simulink library "Lib_Piccolo"  (R2018b)
settings: Solver=VariableStepAuto  StartTime=0.0  StopTime=10.0  RelTol=1e-3
values from neighbouring files (symbols this model uses):
  AccelErrInt2Brakes = 0.15    [SimulationControlConfig16P.m]    (also in SimulationControlConfig16P_F0.m; SimulationControlConfig16P_F2.m; SimulationControlConfig16P_LEGACY.m; SimulationControlConfigTAILLESS.m = 0.2)
  AileronMax = 25    [SimulationControlConfig16P.m]    (also in SimulationControlConfig16P_F0.m; SimulationControlConfig16P_F2.m; SimulationControlConfig16P_LEGACY.m; SimulationControlConfigTAILLESS.m)
  AileronPower = 0.00268    [SimulationControlConfig16P.m]    (also in SimulationControlConfig16P_F0.m; SimulationControlConfig16P_F2.m; SimulationControlConfig16P_LEGACY.m; SimulationControlConfigTAILLESS.m = 0.002266)
  AileronSurfaceMax = 45    [SimulationControlConfig16P.m]    (also in SimulationControlConfig16P_F0.m; SimulationControlConfig16P_F2.m; SimulationControlConfig16P_LEGACY.m; SimulationControlConfigTAILLESS_CGAFT_F0.m = 25)
  AileronTrim = 0    [SimulationControlConfig16P.m]    (also in SimulationControlConfig16P_F0.m; SimulationControlConfig16P_F2.m; SimulationControlConfig16P_LEGACY.m; SimulationControlConfigTAILLESS.m)
  Alt = 1000 + TerrainHeight    [SimulationStateConfig.m]
  AltCruise_m = Alt * 0.3048    [SimulationControlConfig16P.m]    (also in SimulationControlConfig16P_F2.m; SimulationControlConfigTAILLESS.m = Alt/3.28084; SimulationControlConfigTAILLESS_CGAFT_F0.m = 640; SimulationControlConfigTAILLESS_CGFWD_F0.m = 640)
  AltitudeRate2PitchCmdIntegratorInit = 0.1    [SimulationControlPre.m]
  AltMax = 10000    [SimulationControlConfig16P.m]    (also in SimulationControlConfig16P_F0.m; SimulationControlConfig16P_F2.m; SimulationControlConfig16P_LEGACY.m; SimulationControlConfigTAILLESS.m)
  AltMaxAccel = 2.5    [SimulationControlConfig16P.m]    (also in SimulationControlConfig16P_F0.m = 2; SimulationControlConfig16P_F2.m = 2; SimulationControlConfig16P_LEGACY.m = 0.9; SimulationControlConfigTAILLESS.m = 2)
  AltMin = 0    [SimulationControlConfig16P.m]    (also in SimulationControlConfig16P_F0.m; SimulationControlConfig16P_F2.m; SimulationControlConfig16P_LEGACY.m; SimulationControlConfigTAILLESS.m)
  AltRateCmd2Pitch = 0.26    [SimulationControlConfig16P.m]    (also in SimulationControlConfig16P_F0.m = 0.35; SimulationControlConfig16P_F2.m = 0.35; SimulationControlConfig16P_LEGACY.m = 0.6; SimulationControlConfigTAILLESS.m = 0.9)
  AltRateError2Pitch = 0.34    [SimulationControlConfig16P.m]    (also in SimulationControlConfig16P_F0.m = 0.61; SimulationControlConfig16P_F2.m = 0.61; SimulationControlConfig16P_LEGACY.m = 0.4; SimulationControlConfigTAILLESS.m = 0.3)
  AltRateErrorInt2Pitch = 0.61    [SimulationControlConfig16P.m]    (also in SimulationControlConfig16P_F0.m = 0.28; SimulationControlConfig16P_F2.m = 0.28; SimulationControlConfig16P_LEGACY.m = 0.45; SimulationControlConfigTAILLESS.m = 0.15)
  AltRateLpfCutOff = 3    [SimulationControlConfig16P.m]    (also in SimulationControlConfig16P_F0.m; SimulationControlConfig16P_F2.m; SimulationControlConfig16P_LEGACY.m; SimulationControlConfigTAILLESS.m = 5)
  AutoNosegear2Rudder = 26    [SimulationControlConfig16P.m]    (also in SimulationControlConfig16P_F0.m; SimulationControlConfig16P_F2.m; SimulationControlConfig16P_LEGACY.m; SimulationControlConfigTAILLESS.m = 25.2)
  b = 5.54    [SimulationControlConfig16P.m]    (also in SimulationControlConfig16P_F0.m; SimulationControlConfig16P_F2.m; SimulationControlConfig16P_LEGACY.m; SimulationControlConfigTAILLESS.m = 2.37)
  Bank2AileronIntegratorInit = 0    [SimulationControlPre.m]
  BankMax_User = BankMax_User/180*pi    (= 0.610865238198)    [SimulationControlConfig16P.m]    (also in SimulationControlConfig16P_F0.m = 0.523598775598; SimulationControlConfig16P_F2.m = 0.523598775598; SimulationControlConfig16P_LEGACY.m = 0.523598775598; SimulationControlConfigTAILLESS.m = 0.558505360638)
  baseLegFlaps = 20    [SimulationControlConfig16P.m]    (also in SimulationControlConfig16P_F0.m; SimulationControlConfig16P_F2.m = 15; SimulationControlConfig16P_LEGACY.m = 0; SimulationControlConfigTAILLESS.m = 0)
  C = GeneticOpt.C    [SimulationCostFunction.m]
  c = Sw/b    (= 0.841696750903)    [SimulationControlConfig16P.m]    (also in SimulationControlConfig16P_F0.m; SimulationControlConfig16P_F2.m; SimulationControlConfig16P_LEGACY.m; SimulationControlConfigTAILLESS.m = 0.354008438819)
  cell2WheelFactorMG = 5.98    [SimulationSensorConfig16P_LEGACY.m]
  cell2WheelFactorNG = 1    [SimulationSensorConfig16P_LEGACY.m]
  cellSatMaxMG = 15000    [SimulationSensorConfig16P.m]    (also in SimulationSensorConfig16P_LEGACY.m; SimulationSensorConfigTAILLESS7P.m; SimulationSensorConfigUTAIL7P.m)
  cellSatMaxNG = 1000    [SimulationSensorConfig16P.m]    (also in SimulationSensorConfig16P_LEGACY.m; SimulationSensorConfigTAILLESS7P.m; SimulationSensorConfigUTAIL7P.m)
  cellSatMinMG = -15000    [SimulationSensorConfig16P.m]    (also in SimulationSensorConfig16P_LEGACY.m; SimulationSensorConfigTAILLESS7P.m; SimulationSensorConfigUTAIL7P.m)
  cellSatMinNG = -1000    [SimulationSensorConfig16P.m]    (also in SimulationSensorConfig16P_LEGACY.m; SimulationSensorConfigTAILLESS7P.m; SimulationSensorConfigUTAIL7P.m)
  CL_Limit = CL_Max    (= 0.54)    [SimulationControlConfig16P.m]    (also in SimulationControlConfig16P_F0.m; SimulationControlConfig16P_F2.m = 0.638; SimulationControlConfig16P_LEGACY.m; SimulationControlConfigTAILLESS.m = 0.525)
  CL_Max = 0.54    [SimulationControlConfig16P.m]    (also in SimulationControlConfig16P_F0.m; SimulationControlConfig16P_F2.m = 0.638; SimulationControlConfig16P_LEGACY.m; SimulationControlConfigTAILLESS.m = 0.525)
  CL_Max_Nom = 0.465    [SimulationControlConfig16P.m]    (also in SimulationControlConfig16P_F0.m; SimulationControlConfig16P_F2.m = 0.563; SimulationControlConfig16P_LEGACY.m; SimulationControlConfigTAILLESS.m = 0.39)
  CL_Min = 0    [SimulationControlConfig16P.m]    (also in SimulationControlConfig16P_F0.m; SimulationControlConfig16P_F2.m; SimulationControlConfig16P_LEGACY.m; SimulationControlConfigTAILLESS.m)
  ClimbMaxFraction = 0.35    [SimulationControlConfig16P.m]    (also in SimulationControlConfig16P_F0.m = 0.17; SimulationControlConfig16P_F2.m = 0.17; SimulationControlConfig16P_LEGACY.m = 0.24; SimulationControlConfigTAILLESS.m = 0.21)
  ClimboutMaxBank = 7.0    (= 7)    [SimulationControlConfig16P.m]    (also in SimulationControlConfig16P_F0.m; SimulationControlConfig16P_F2.m; SimulationControlConfig16P_LEGACY.m; SimulationControlConfigTAILLESS.m = 5)
  ClimboutTimer = 7.0    (= 7)    [SimulationControlConfig16P.m]    (also in SimulationControlConfig16P_F0.m; SimulationControlConfig16P_F2.m; SimulationControlConfig16P_LEGACY.m; SimulationControlConfigTAILLESS.m)
  dCl_per_dFlap = 0.005581818    [SimulationControlConfig16P.m]    (also in SimulationControlConfig16P_F0.m = 0; SimulationControlConfig16P_F2.m = 0.0065; SimulationControlConfig16P_LEGACY.m = 0; SimulationControlConfigTAILLESS.m = 0)
  DecelerationCmd = 3.1    [SimulationControlConfig16P.m]    (also in SimulationControlConfig16P_F0.m; SimulationControlConfig16P_F2.m; SimulationControlConfig16P_LEGACY.m; SimulationControlConfigTAILLESS.m = 0.1)
  DeRotateLogicEndTimer = abs((NoseDownLimit_Deg-1)/DeRotateRamp_Dps)    [SimulationControlConfig16P.m]    (also in SimulationControlConfig16P_F0.m; SimulationControlConfig16P_F2.m; SimulationControlConfig16P_LEGACY.m; SimulationControlConfigTAILLESS.m)
  DeRotateLogicHoldNoseUpTimer = 0.1    [SimulationControlConfig16P.m]    (also in SimulationControlConfig16P_F0.m; SimulationControlConfig16P_F2.m; SimulationControlConfig16P_LEGACY.m; SimulationControlConfigTAILLESS.m)
  DeRotateLogicTimerTimeout = 2    [SimulationControlConfig16P.m]    (also in SimulationControlConfig16P_F0.m; SimulationControlConfig16P_F2.m; SimulationControlConfig16P_LEGACY.m; SimulationControlConfigTAILLESS.m)
  DeRotateLowerCmdSaturation = 0    [SimulationControlConfig16P.m]    (also in SimulationControlConfig16P_F0.m; SimulationControlConfig16P_F2.m; SimulationControlConfig16P_LEGACY.m; SimulationControlConfigTAILLESS.m)
  DeRotateRamp_Dps = 3    [SimulationControlConfig16P.m]    (also in SimulationControlConfig16P_F0.m; SimulationControlConfig16P_F2.m; SimulationControlConfig16P_LEGACY.m; SimulationControlConfigTAILLESS.m = 8)
  DeRotateUpperCmdSaturation = 7    [SimulationControlConfig16P.m]    (also in SimulationControlConfig16P_F0.m; SimulationControlConfig16P_F2.m; SimulationControlConfig16P_LEGACY.m; SimulationControlConfigTAILLESS.m)
  DescentMaxFraction = 0.22    [SimulationControlConfig16P.m]    (also in SimulationControlConfig16P_F0.m = 0.2; SimulationControlConfig16P_F2.m = 0.2; SimulationControlConfig16P_LEGACY.m = 0.2; SimulationControlConfigTAILLESS.m = 0.17)
  DesktopSimTerrainOffset_m = 0.406    [SimulationAircraftConfig.m]
  downwindFlaps = 0    [SimulationControlConfig16P.m]    (also in SimulationControlConfig16P_F0.m; SimulationControlConfig16P_F2.m = 15; SimulationControlConfig16P_LEGACY.m; SimulationControlConfigTAILLESS.m)
  downwindSplitAil = 0    [SimulationControlConfig16P_F2.m]
  DP_init = 0.5*1.225*V_init^2    [SimulationControlConfig16P.m]    (also in SimulationControlConfig16P_F0.m; SimulationControlConfig16P_F2.m; SimulationControlConfig16P_LEGACY.m; SimulationControlConfigTAILLESS.m)
  dscNoiseMG = 1    [SimulationSensorConfig16P_LEGACY.m]
  dscNoiseNG = 0.25    [SimulationSensorConfig16P_LEGACY.m]
  DSCnumBits = 24    [SimulationSensorConfig16P.m]    (also in SimulationSensorConfig16P_LEGACY.m; SimulationSensorConfigTAILLESS7P.m; SimulationSensorConfigUTAIL7P.m)
  DSCRangeMaxMG = 15000    [SimulationSensorConfig16P.m]    (also in SimulationSensorConfig16P_LEGACY.m; SimulationSensorConfigTAILLESS7P.m; SimulationSensorConfigUTAIL7P.m)
  DSCRangeMaxNG = 1000    [SimulationSensorConfig16P.m]    (also in SimulationSensorConfig16P_LEGACY.m; SimulationSensorConfigTAILLESS7P.m; SimulationSensorConfigUTAIL7P.m)
  DSCRangeMinMG = -15000    [SimulationSensorConfig16P.m]    (also in SimulationSensorConfig16P_LEGACY.m; SimulationSensorConfigTAILLESS7P.m; SimulationSensorConfigUTAIL7P.m)
  DSCRangeMinNG = -1000    [SimulationSensorConfig16P.m]    (also in SimulationSensorConfig16P_LEGACY.m; SimulationSensorConfigTAILLESS7P.m; SimulationSensorConfigUTAIL7P.m)
  dt = DLLSim.dt    [SimulationTimeStep.m]    (also in SimulationTrim.m = 0.02)
  EarlyTouchdownThreshold = 3.0    (= 3)    [SimulationControlConfig16P.m]    (also in SimulationControlConfig16P_F0.m; SimulationControlConfig16P_F2.m; SimulationControlConfig16P_LEGACY.m; SimulationControlConfigTAILLESS.m)
  ElevatorDeflectionRate = 15    [SimulationControlConfig16P.m]    (also in SimulationControlConfig16P_F0.m; SimulationControlConfig16P_F2.m; SimulationControlConfig16P_LEGACY.m = 12; SimulationControlConfigTAILLESS.m = 5)
  ElevatorMax = 25    [SimulationControlConfig16P.m]    (also in SimulationControlConfig16P_F0.m; SimulationControlConfig16P_F2.m; SimulationControlConfig16P_LEGACY.m; SimulationControlConfigTAILLESS.m)
  ElevatorPower = -0.002209    [SimulationControlConfig16P.m]    (also in SimulationControlConfig16P_F0.m; SimulationControlConfig16P_F2.m; SimulationControlConfig16P_LEGACY.m; SimulationControlConfigTAILLESS.m = -0.002668)
  ElevatorTrim = -3.5    [SimulationControlConfig16P.m]    (also in SimulationControlConfig16P_F0.m; SimulationControlConfig16P_F2.m; SimulationControlConfig16P_LEGACY.m; SimulationControlConfigTAILLESS.m = -3)
  elevonBias = 0    [SimulationControlConfig16P.m]    (also in SimulationControlConfig16P_F0.m; SimulationControlConfig16P_F2.m; SimulationControlConfig16P_LEGACY.m; SimulationControlConfigTAILLESS.m)
  Enable_TAS_Protection = 0    [SimulationControlConfig16P.m]    (also in SimulationControlConfig16P_F0.m; SimulationControlConfig16P_F2.m; SimulationControlConfig16P_LEGACY.m; SimulationControlConfigTAILLESS.m)
  EnableCrossTrackAbort = 1    [SimulationControlConfig16P.m]    (also in SimulationControlConfigTAILLESS.m; SimulationControlConfigTAILLESS_CGAFT_F0.m; SimulationControlConfigTAILLESS_CGFWD_F0.m; SimulationControlConfigTAILLESS_CGFWD_F2.m)
  EnergyBandwidth = 0.04    [SimulationControlConfig16P.m]    (also in SimulationControlConfig16P_F0.m = 0.03; SimulationControlConfig16P_F2.m = 0.03; SimulationControlConfig16P_LEGACY.m = 0.02; SimulationControlConfigTAILLESS.m = 0.06)
  EngineLhFuelCut = 0    [SimulationAircraftConfig.m]
  EngineRhFuelCut = 0    [SimulationAircraftConfig.m]
  FastThrottleRate = 0.075    [SimulationControlConfig16P.m]    (also in SimulationControlConfig16P_F0.m = 0.05; SimulationControlConfig16P_F2.m = 0.05; SimulationControlConfig16P_LEGACY.m = 0.05; SimulationControlConfigTAILLESS.m = 0.1)
  FilterWarmUpTime = 2    [SimulationSensorConfig16P.m]    (also in SimulationSensorConfig16P_LEGACY.m; SimulationSensorConfigTAILLESS7P.m; SimulationSensorConfigUTAIL7P.m)
  finalApproachFlaps = 20    [SimulationControlConfig16P.m]    (also in SimulationControlConfig16P_F0.m; SimulationControlConfig16P_F2.m = 15; SimulationControlConfig16P_LEGACY.m = 0; SimulationControlConfigTAILLESS.m = 0)
  finalApproachSplitAil = 20    [SimulationControlConfig16P_F2.m]
  FinalDescentSlope_Deg = testPlans(testIndx).descentSlope    [SimulationControlConfig16P.m]    (also in SimulationControlConfig16P_F0.m; SimulationControlConfig16P_F2.m; SimulationControlConfig16P_LEGACY.m; SimulationControlConfigTAILLESS.m)
  flapMax = 0    [SimulationControlConfig16P.m]    (also in SimulationControlConfig16P_F0.m = 35; SimulationControlConfig16P_F2.m = 33; SimulationControlConfig16P_LEGACY.m; SimulationControlConfigTAILLESS.m)
  flapRate = 7.5    [SimulationControlConfig16P.m]    (also in SimulationControlConfig16P_F0.m; SimulationControlConfig16P_F2.m; SimulationControlConfig16P_LEGACY.m; SimulationControlConfigTAILLESS.m = 6.6)
  FlareHeight = 5    [SimulationControlConfig16P.m]    (also in SimulationControlConfig16P_F0.m; SimulationControlConfig16P_F2.m; SimulationControlConfig16P_LEGACY.m = 4.8; SimulationControlConfigTAILLESS.m = 2.75)
  FlareVerticalRate_mps = -0.4    [SimulationControlConfig16P.m]    (also in SimulationControlConfig16P_F0.m; SimulationControlConfig16P_F2.m; SimulationControlConfig16P_LEGACY.m = -0.5; SimulationControlConfigTAILLESS.m = -0.15)
  Fp_Aileron = 0.55*2*pi*RollRateLpfCutoff*dt    [SimulationControlConfig16P.m]    (also in SimulationControlConfig16P_F0.m; SimulationControlConfig16P_F2.m; SimulationControlConfig16P_LEGACY.m; SimulationControlConfigTAILLESS.m)
  Fp_Alt = 2*pi*0.55*AltBandwidth    (= 0.622035345411)    [SimulationControlConfig16P.m]    (also in SimulationControlConfig16P_F0.m; SimulationControlConfig16P_F2.m; SimulationControlConfig16P_LEGACY.m = 0.099; SimulationControlConfigTAILLESS.m = 0.207345115137)
  Fp_AltRate = 0.55*2*pi*AltRateLpfCutOff*dt    [SimulationControlConfig16P.m]    (also in SimulationControlConfig16P_F0.m; SimulationControlConfig16P_F2.m; SimulationControlConfig16P_LEGACY.m; SimulationControlConfigTAILLESS.m)
  Fp_Elevator = 0.55*2*pi*PitchRateLpfCutoff*dt    [SimulationControlConfig16P.m]    (also in SimulationControlConfig16P_F0.m; SimulationControlConfig16P_F2.m; SimulationControlConfig16P_LEGACY.m; SimulationControlConfigTAILLESS.m)
  Fp_Energy = 0.55*2*pi*EnergyBandwidth    (= 0.138230076758)    [SimulationControlConfig16P.m]    (also in SimulationControlConfig16P_F0.m = 0.103672557568; SimulationControlConfig16P_F2.m = 0.103672557568; SimulationControlConfig16P_LEGACY.m = 0.069115038379; SimulationControlConfigTAILLESS.m = 0.207345115137)
  Fp_Energy2 = 0.55*2*pi*EnergyBandwidth*dt    [SimulationControlConfig16P.m]    (also in SimulationControlConfig16P_F0.m; SimulationControlConfig16P_F2.m; SimulationControlConfig16P_LEGACY.m; SimulationControlConfigTAILLESS.m)
  Fp_Pitch = 0.55*2*pi*PitchBandwidth    (= 2.45358386245)    [SimulationControlConfig16P.m]    (also in SimulationControlConfig16P_F0.m; SimulationControlConfig16P_F2.m = 1.72787595947; SimulationControlConfig16P_LEGACY.m = 3.11017672705; SimulationControlConfigTAILLESS.m = 1.55508836353)
  Fp_Pitch_2 = 0.55*2*pi*PitchBandwidth*dt    [SimulationControlConfig16P.m]    (also in SimulationControlConfig16P_F0.m; SimulationControlConfig16P_F2.m; SimulationControlConfig16P_LEGACY.m; SimulationControlConfigTAILLESS.m)
  Fp_Roll = RollBandwidth^2    (= 1.69)    [SimulationControlConfig16P.m]    (also in SimulationControlConfig16P_F0.m = 1.44; SimulationControlConfig16P_F2.m = 1.44; SimulationControlConfig16P_LEGACY.m = 1.44; SimulationControlConfigTAILLESS.m = 1.21)
  Fp_Rudder = 0.55*2*pi*YawRateLpfCutoff*dt    [SimulationControlConfig16P.m]    (also in SimulationControlConfig16P_F0.m; SimulationControlConfig16P_F2.m; SimulationControlConfig16P_LEGACY.m; SimulationControlConfigTAILLESS.m)
  Fp_TAS = 0.55*2*pi*TASBandwidth    (= 0.103672557568)    [SimulationControlConfig16P.m]    (also in SimulationControlConfig16P_F0.m; SimulationControlConfig16P_F2.m; SimulationControlConfig16P_LEGACY.m; SimulationControlConfigTAILLESS.m = 0.172787595947)
  Fp_TAS_Filter = 2*pi*TasLpfCutoff*dt    [SimulationControlConfig16P.m]    (also in SimulationControlConfig16P_F0.m; SimulationControlConfig16P_F2.m; SimulationControlConfig16P_LEGACY.m; SimulationControlConfigTAILLESS.m)
  Fp_Turn = 0.55*2*pi*TurnErrLPFcutoff    (= 0.172787595947)    [SimulationControlConfig16P.m]    (also in SimulationControlConfig16P_F0.m = 0.0345575191895; SimulationControlConfig16P_F2.m = 0.0345575191895; SimulationControlConfig16P_LEGACY.m = 0.0345575191895; SimulationControlConfigTAILLESS.m)
  Fp_TurnDerr = 0.55*2*pi*TurnDerivativeLPFcutoff    (= 0.172787595947)    [SimulationControlConfig16P.m]    (also in SimulationControlConfig16P_F0.m = 0.0345575191895; SimulationControlConfig16P_F2.m = 0.0345575191895; SimulationControlConfig16P_LEGACY.m = 0.0345575191895; SimulationControlConfigTAILLESS.m)
  FTV = 3    [SimulationAircraftConfig.m]
  ftvStaticPositionError = 1/1.18    (= 0.847457627119)    [SimulationSensorConfig16P.m]    (also in SimulationSensorConfig16P_LEGACY.m; SimulationSensorConfigTAILLESS7P.m = 1; SimulationSensorConfigUTAIL7P.m = 1)
  g = 9.81    [SimulationStateConfig.m]
  goAroundSplitAil = 0    [SimulationControlConfig16P_F2.m]
  GustSpd_Kts = testPlans(testIndx).gustSpd    [SimulationStateConfig.m]
  GustTriggerVal = testPlans(testIndx).gustTriggerVal    [SimulationStateConfig.m]
  HeadingErr2TurnRate = 0.5    [SimulationControlConfig16P.m]    (also in SimulationControlConfig16P_F0.m; SimulationControlConfig16P_F2.m; SimulationControlConfig16P_LEGACY.m; SimulationControlConfigTAILLESS.m)
  HeadingErrDer2TurnRate = 0.3    [SimulationControlConfig16P.m]    (also in SimulationControlConfig16P_F0.m; SimulationControlConfig16P_F2.m; SimulationControlConfig16P_LEGACY.m; SimulationControlConfigTAILLESS.m)
  IASbounce = IASstall*0.8    [SimulationControlPre.m]
  IAScruiseCMD = sqrt(2*m*9.81/(1.225*Sw*CL_cruise))    [SimulationControlConfig16P.m]    (also in SimulationControlConfig16P_F0.m; SimulationControlConfig16P_F2.m; SimulationControlConfig16P_LEGACY.m; SimulationControlConfigTAILLESS.m)
  IASfinalCMD = 1.12 * IASmin    [SimulationControlConfig16P.m]    (also in SimulationControlConfig16P_F0.m = 1.14 * IASmin; SimulationControlConfig16P_F2.m = 1.10 * IASmin; SimulationControlConfig16P_LEGACY.m = 1.10 * IASmin; SimulationControlConfigTAILLESS.m = 1.14 * IASmin)
  IASflareCMD = IASstall    [SimulationControlConfig16P.m]    (also in SimulationControlConfig16P_F0.m; SimulationControlConfig16P_F2.m; SimulationControlConfig16P_LEGACY.m; SimulationControlConfigTAILLESS.m)
  IASmax = 64    [SimulationControlConfig16P.m]    (also in SimulationControlConfig16P_F0.m = 46; SimulationControlConfig16P_F2.m = 52; SimulationControlConfig16P_LEGACY.m = 46; SimulationControlConfigTAILLESS.m = 38.9)
  IASmin = sqrt(2*m*9.81/(1.225*Sw*0.9*CL_Max_Nom))    [SimulationControlConfig16P.m]    (also in SimulationControlConfig16P_F0.m; SimulationControlConfig16P_F2.m; SimulationControlConfig16P_LEGACY.m; SimulationControlConfigTAILLESS.m)
  IASshortCMD = IASstall    [SimulationControlConfig16P.m]    (also in SimulationControlConfig16P_F0.m; SimulationControlConfig16P_F2.m; SimulationControlConfig16P_LEGACY.m; SimulationControlConfigTAILLESS.m)
  IASstall = sqrt(2*m*9.81/(1.225*Sw*CL_Max))    [SimulationControlConfig16P.m]    (also in SimulationControlConfig16P_F0.m; SimulationControlConfig16P_F2.m; SimulationControlConfig16P_LEGACY.m; SimulationControlConfigTAILLESS.m)
  inFlight = 1    [SimulationControlConfig16P.m]    (also in SimulationControlConfigTAILLESS.m; SimulationControlConfigTAILLESS_CGAFT_F0.m; SimulationControlConfigTAILLESS_CGFWD_F0.m; SimulationControlConfigTAILLESS_CGFWD_F2.m)
  JetCatOffset = 5    [SimulationControlConfig16P.m]    (also in SimulationControlConfig16P_F0.m; SimulationControlConfig16P_F2.m; SimulationControlConfig16P_LEGACY.m)
  LaunchRollingElevator = -1.5    [SimulationControlConfig16P.m]    (also in SimulationControlConfig16P_F0.m; SimulationControlConfig16P_F2.m = 1.25; SimulationControlConfig16P_LEGACY.m; SimulationControlConfigTAILLESS.m = 1)
  ldg_NosegearMax = 10    [SimulationControlConfig16P.m]    (also in SimulationControlConfig16P_F0.m; SimulationControlConfig16P_F2.m; SimulationControlConfig16P_LEGACY.m; SimulationControlConfigTAILLESS.m)
  ldg_TrackVyErrInt2Nosegear = 0.1250    (= 0.125)    [SimulationControlConfig16P.m]    (also in SimulationControlConfig16P_F0.m; SimulationControlConfig16P_F2.m; SimulationControlConfig16P_LEGACY.m; SimulationControlConfigTAILLESS.m = 0.00714285714286)
  ldg_TrackVyErrPro2Nosegear = 0.35    [SimulationControlConfig16P.m]    (also in SimulationControlConfig16P_F0.m; SimulationControlConfig16P_F2.m; SimulationControlConfig16P_LEGACY.m; SimulationControlConfigTAILLESS.m = 0.0546666666667)
  ldg_TrackY2Vy = 0.07    [SimulationControlConfig16P.m]    (also in SimulationControlConfig16P_F0.m; SimulationControlConfig16P_F2.m; SimulationControlConfig16P_LEGACY.m; SimulationControlConfigTAILLESS.m = 0.17)
  ldg_Vy2NosegearScalingPower = 1.075    [SimulationControlConfig16P.m]    (also in SimulationControlConfig16P_F0.m; SimulationControlConfig16P_F2.m; SimulationControlConfig16P_LEGACY.m; SimulationControlConfigTAILLESS.m = 0.6)
  ldg_Y2VyScalingPower = 0.175    [SimulationControlConfig16P.m]    (also in SimulationControlConfig16P_F0.m; SimulationControlConfig16P_F2.m; SimulationControlConfig16P_LEGACY.m; SimulationControlConfigTAILLESS.m = 0)
  ldg_YawRate2Nosegear = 0.175    [SimulationControlConfig16P.m]    (also in SimulationControlConfig16P_F0.m; SimulationControlConfig16P_F2.m; SimulationControlConfig16P_LEGACY.m; SimulationControlConfigTAILLESS.m = 0.065)
  LiftSlope = 0.064285    [SimulationControlConfig16P.m]    (also in SimulationControlConfig16P_F0.m; SimulationControlConfig16P_F2.m; SimulationControlConfig16P_LEGACY.m; SimulationControlConfigTAILLESS.m = 0.058631)
  LPFaileronInit = 0    [SimulationControlPre.m]
  LPFclestInit = 0    [SimulationControlPre.m]
  LPFenergyFFInit = 0    [SimulationControlPre.m]
  ... (+122 more)
undefined symbols (not defined in the file or in its folder): abortFlag, alphaHPF, apmDelay, BRWNOUT, CRAWOR, CRAWUR, DiscIntNeverNeededParam, DLLSim, DLLSimStep, ECOMOR, ECOMUR, Fp_Tas, GustTrigger_HeightAgl_m, IPSTAT, LCINTEG, Ldg_Persist_Time, LOWER_FLAGS, MSG_ENABLE, NoiseStd, OLDVAL, OVERRIDE_ENABLE, OVERRIDE_VALUE, REBOOT, reversionEnable, revIASMax, revIASMin, revPitchMax, revPitchMin, revPitchRateMax, revRollMax, revRollRateMax, SAMPLE, SCALON, SensorModel, sigbuilder_block, Sim_Vx, Sim_Vy, Sim_Vz, Sim_Xpos, Sim_Ypos, Sim_Zpos, SYSOR, SYSUR, TARE, TEMPOR, TEMPUR, testIndx, testPlan, testPlans, Trim_piccoloInCmd, Trim_REFSI_FD_IN_nmodeCgShifterCmd_Flag, Trim_REFSI_FD_IN_nmodeCgShifterCmd_Ft, Trim_REFSI_FD_IN_nmodeCgShifterCmdType, Trim_REFSI_FD_IN_nmodeCgShifterNRCActive, Trim_REFSI_FD_IN_nmodeFlapLhIBCmd_Deg, Trim_REFSI_FD_IN_nmodeFlapLhOBCmd_Deg, Trim_REFSI_FD_IN_nmodeFlapRhIBCmd_Deg, Trim_REFSI_FD_IN_nmodeFlapRhOBCmd_Deg, Trim_REFSI_FD_IN_nmodeSlatLhCmd_Deg ... (+11)
libraries: simulink x1237, $bdroot x179, aerolibconvert2 x63, dspswit3 x25, aerolibatmos2 x5, simulink_extras x4, dsparch4 x2, Lib_Piccolo_Alt x2, eeGeneralControl x1, dspindex x1
(part 35 of 74)

== system Lib_Piccolo/Ground Detection Systems/WoW Wrapper/Variant Subsystem/Load Cell WoW Model 21 ==
  note: K2 System Boundary
  note: Wheel loads from FDM, units of lbf .
  note: CANOpen transport delay from DSC to K2 is <1ms. Addtional delay here also accounts for worst case asynchronicity between DSC PDO and K2 sampling. Load phase delay defined in workspace.
  note: Data Formatting for Piccolo Communications
  note: K2 Data Acquisition and Processing
  note: DSC Model
  note: Load Cell Model
  note: These signals are sent on the CMD and TELEM CAN Bus in the 0x3280000 ID Message
  note: This subsystem is auto-coded to generate the WOW class as integrated by K2. Inports and Outports defined here will constitute the class interface.
  note: Calibrated/converted Wheel loads, as used by WOW logic, units of N .
      |
      | This subsystem is auto-coded and implements signal conditioning of loads prior to use in WOW logic. Inports and Outports defined here will constitute the class interface.
  note: Converted to Cell loads, units of N .
  note: Quantized DSC loads, units of N .
  Piccolo_AP_Mode : Inport
  Bus Element In5 : Inport  Port=2  PortName=WoW_Bus_In  Element=ZgrndRhLbs
  Bus Element In4 : Inport  Port=2  PortName=WoW_Bus_In  Element=ZgrndLhLbs
  Bus Element In1 : Inport  Port=2  PortName=WoW_Bus_In  Element=ZgrndNgLbs
  Bus Creator : BusCreator  Inputs=2
  Bus Selector : BusSelector  OutputSignals=CONTACT
  Bus Formatting MGL : Subsystem
  Bus Formatting MGR : Subsystem
  Bus Formatting NG : Subsystem
  Constant1 : Constant  Value=0  OutDataTypeStr=boolean
  Constant3 : Constant  Value=0  OutDataTypeStr=boolean
  DSC Data Acquisition : Subsystem
  DSC Load Conversion : $bdroot/DSC Load Conversion  SystemSampleTime=-1
  Data Type Conversion : DataTypeConversion
  Data Type Conversion1 : DataTypeConversion
  Data Type Conversion2 : DataTypeConversion  OutDataTypeStr=uint8
  Delay1 : Delay  DelayLength=SensorModel.WOW.Cell.WOWtransportDelay
  Delay2 : Delay  DelayLength=SensorModel.WOW.Cell.WOWtransportDelay
  Delay3 : Delay  DelayLength=SensorModel.WOW.Cell.WOWtransportDelay
  Gain : Gain  Gain=100
  Load Cell and Unit Conversion : Subsystem
  Re-Encoding L : Quantizer  QuantizationInterval=(SensorModel.WOW.Cell.satMaxMG-SensorModel.WOW.Cell.satMinMG)/(2^SensorModel.WOW.Cell.numBits)
  Re-Encoding N : Quantizer  QuantizationInterval=(SensorModel.WOW.Cell.satMaxNG-SensorModel.WOW.Cell.satMinNG)/(2^SensorModel.WOW.Cell.numBits)
  Re-Encoding R : Quantizer  QuantizationInterval=(SensorModel.WOW.Cell.satMaxMG-SensorModel.WOW.Cell.satMinMG)/(2^SensorModel.WOW.Cell.numBits)  LinearizeAsGain=off
  Saturation L : Saturate  UpperLimit=SensorModel.WOW.Cell.satMaxMG  LowerLimit=SensorModel.WOW.Cell.satMinMG
  Saturation N : Saturate  UpperLimit=SensorModel.WOW.Cell.satMaxNG  LowerLimit=SensorModel.WOW.Cell.satMinNG
  Saturation R : Saturate  UpperLimit=SensorModel.WOW.Cell.satMaxMG  LowerLimit=SensorModel.WOW.Cell.satMinMG
  Signal Specification L : SignalSpecification  OutDataTypeStr=single  Dimensions=[1 1]  SampleTime=dt
  Signal Specification N : SignalSpecification  OutDataTypeStr=single  Dimensions=[1 1]  SampleTime=dt
  Signal Specification R : SignalSpecification  OutDataTypeStr=single  Dimensions=[1 1]  SampleTime=dt
  Subsystem : Subsystem
  Terminator{,1..10} (11 alike) : Terminator
  WOW Module : Subsystem
  WOW_Bus_Out : Outport
  tag scope: Sim_WOW_Output_Disable=global
  wires:
  Piccolo_AP_Mode/1 -> WOW Module/1(PICCOLO_AP_MODE)
  Signal Specification R/1 -> Saturation R/1, DSC Load Conversion/3  "Sim.MGR_DSC_Load_N"
  Signal Specification L/1 -> Saturation L/1, DSC Load Conversion/2  "Sim.MGL_DSC_Load_N"
  Signal Specification N/1 -> DSC Load Conversion/1, Saturation N/1  "Sim.NG_DSC_Load_N"
  Bus Selector/1 -> Data Type Conversion2/1  "<CONTACT>"
  Bus Creator/1 -> WOW_Bus_Out/1
  Data Type Conversion/1 -> Bus Creator/1  "ContactBool"
  Gain/1 -> Data Type Conversion1/1
  Data Type Conversion1/1 -> Bus Creator/2  "WoWPcnt"
  Delay1/1 -> Signal Specification L/1
  Delay2/1 -> Signal Specification R/1
  Delay3/1 -> Signal Specification N/1
  Re-Encoding R/1 -> Terminator10/1  "Sim.328_MGR_DSC_Load_N"
  Re-Encoding L/1 -> Terminator9/1  "Sim.328_MGL_DSC_Load_N"
  Re-Encoding N/1 -> Terminator/1  "Sim.328_NG_DSC_Load_N"
  WOW Module/2(WOW_OUTPUT_DISABLE) -> [Sim_WOW_Output_Disable]
  Data Type Conversion2/1 -> Gain/1, Data Type Conversion/1
  Constant3/1 -> WOW Module/2(NRC_ACTIVE)
  Constant1/1 -> WOW Module/6(INITIALIZE)
  Subsystem/1(User Cmds) -> WOW Module/7(User_Cmd_In)
  WOW Module/1(Detection) -> Bus Selector/1
  WOW Module/3(NG_Out) -> Terminator1/1
  WOW Module/5(MGR_Out) -> Terminator2/1
  WOW Module/4(MGL_Out) -> Terminator3/1
  WOW Module/6(SHY_MODE) -> Terminator4/1
  WOW Module/7(User_Cmd_Out) -> Terminator5/1
  Bus Formatting NG/1(Bus Out) -> WOW Module/3(NG_In)
  Bus Formatting MGL/1(Bus Out) -> WOW Module/4(MGL_In)
  Bus Formatting MGR/1(Bus Out) -> WOW Module/5(MGR_In)
  DSC Load Conversion/1 -> Bus Formatting NG/1(WOW_N)  "Sim.NG_WOW_N"
  DSC Load Conversion/3 -> Bus Formatting MGL/1(WOW_N)  "Sim.MGL_WOW_N"
  DSC Load Conversion/5 -> Bus Formatting MGR/1(WOW_N)  "Sim.MGR_WOW_N"
  Saturation N/1 -> Re-Encoding N/1
  Saturation L/1 -> Re-Encoding L/1
  Saturation R/1 -> Re-Encoding R/1
  Bus Element In1/1 -> Load Cell and Unit Conversion/1(NG Wheel Load Lbf)
  Bus Element In4/1 -> Load Cell and Unit Conversion/2(MGL Wheel Load Lbf)
  Bus Element In5/1 -> Load Cell and Unit Conversion/3(MGR Wheel Load Lbf)
  Load Cell and Unit Conversion/1(NG Cell Load N) -> DSC Data Acquisition/1(NG Cell Load N)
  Load Cell and Unit Conversion/2(MGL Cell Load N) -> DSC Data Acquisition/2(MGL Cell Load N)
  Load Cell and Unit Conversion/3(MGR Cell Load N) -> DSC Data Acquisition/3(MGR Cell Load N)
  DSC Data Acquisition/1(NG DSC Load N) -> Delay3/1
  DSC Data Acquisition/2(MGL DSC Load N) -> Delay1/1
  DSC Data Acquisition/3(MGR DSC Load N) -> Delay2/1
  DSC Load Conversion/2 -> Terminator6/1
  DSC Load Conversion/4 -> Terminator7/1
  DSC Load Conversion/6 -> Terminator8/1

== system Lib_Piccolo/Ground Detection Systems/WoW Wrapper/Variant Subsystem/Load Cell WoW Model 22 ==
  note: K2 System Boundary
  note: Wheel loads from FDM, units of lbf .
  note: CANOpen transport delay from DSC to K2 is <1ms. Addtional delay here also accounts for worst case asynchronicity between DSC PDO and K2 sampling. Load phase delay defined in workspace.
  note: Data Formatting for Piccolo Communications
  note: K2 Data Acquisition and Processing
  note: DSC Model
  note: Load Cell Model
  note: These signals are sent on the CMD and TELEM CAN Bus in the 0x3280000 ID Message
  note: This subsystem is auto-coded to generate the WOW class as integrated by K2. Inports and Outports defined here will constitute the class interface.
  note: Calibrated/converted Wheel loads, as used by WOW logic, units of N .
      |
      | This subsystem is auto-coded and implements signal conditioning of loads prior to use in WOW logic. Inports and Outports defined here will constitute the class interface.
  note: Converted to Cell loads, units of N .
  note: Quantized DSC loads, units of N .
  Piccolo_AP_Mode : Inport
  Bus Element In5 : Inport  Port=2  PortName=WoW_Bus_In  Element=ZgrndRhLbs
  Bus Element In4 : Inport  Port=2  PortName=WoW_Bus_In  Element=ZgrndLhLbs
  Bus Element In1 : Inport  Port=2  PortName=WoW_Bus_In  Element=ZgrndNgLbs
  Bus Creator : BusCreator  Inputs=2
  Bus Selector : BusSelector  OutputSignals=CONTACT
  Bus Formatting MGL : Subsystem
  Bus Formatting MGR : Subsystem
  Bus Formatting NG : Subsystem
  Constant1 : Constant  Value=0  OutDataTypeStr=boolean
  Constant3 : Constant  Value=0  OutDataTypeStr=boolean
  DSC Data Acquisition : Subsystem
  DSC Load Conversion : $bdroot/DSC Load Conversion  SystemSampleTime=-1
  Data Type Conversion : DataTypeConversion
  Data Type Conversion1 : DataTypeConversion
  Data Type Conversion2 : DataTypeConversion  OutDataTypeStr=uint8
  Delay1 : Delay  DelayLength=SensorModel.WOW.Cell.WOWtransportDelay
  Delay2 : Delay  DelayLength=SensorModel.WOW.Cell.WOWtransportDelay
  Delay3 : Delay  DelayLength=SensorModel.WOW.Cell.WOWtransportDelay
  Gain : Gain  Gain=100
  Load Cell and Unit Conversion : Subsystem
  Re-Encoding L : Quantizer  QuantizationInterval=(SensorModel.WOW.Cell.satMaxMG-SensorModel.WOW.Cell.satMinMG)/(2^SensorModel.WOW.Cell.numBits)
  Re-Encoding N : Quantizer  QuantizationInterval=(SensorModel.WOW.Cell.satMaxNG-SensorModel.WOW.Cell.satMinNG)/(2^SensorModel.WOW.Cell.numBits)
  Re-Encoding R : Quantizer  QuantizationInterval=(SensorModel.WOW.Cell.satMaxMG-SensorModel.WOW.Cell.satMinMG)/(2^SensorModel.WOW.Cell.numBits)  LinearizeAsGain=off
  Saturation L : Saturate  UpperLimit=SensorModel.WOW.Cell.satMaxMG  LowerLimit=SensorModel.WOW.Cell.satMinMG
  Saturation N : Saturate  UpperLimit=SensorModel.WOW.Cell.satMaxNG  LowerLimit=SensorModel.WOW.Cell.satMinNG
  Saturation R : Saturate  UpperLimit=SensorModel.WOW.Cell.satMaxMG  LowerLimit=SensorModel.WOW.Cell.satMinMG
  Signal Specification L : SignalSpecification  OutDataTypeStr=single  Dimensions=[1 1]  SampleTime=dt
  Signal Specification N : SignalSpecification  OutDataTypeStr=single  Dimensions=[1 1]  SampleTime=dt
  Signal Specification R : SignalSpecification  OutDataTypeStr=single  Dimensions=[1 1]  SampleTime=dt
  Subsystem : Subsystem
  Terminator{,1..10} (11 alike) : Terminator
  WOW Module : Subsystem
  WOW_Bus_Out : Outport
  tag scope: Sim_WOW_Output_Disable=global
  wires:
  Piccolo_AP_Mode/1 -> WOW Module/1(PICCOLO_AP_MODE)
  Signal Specification R/1 -> Saturation R/1, DSC Load Conversion/3  "Sim.MGR_DSC_Load_N"
  Signal Specification L/1 -> Saturation L/1, DSC Load Conversion/2  "Sim.MGL_DSC_Load_N"
  Signal Specification N/1 -> DSC Load Conversion/1, Saturation N/1  "Sim.NG_DSC_Load_N"
  Bus Selector/1 -> Data Type Conversion2/1  "<CONTACT>"
  Bus Creator/1 -> WOW_Bus_Out/1
  Data Type Conversion/1 -> Bus Creator/1  "ContactBool"
  Gain/1 -> Data Type Conversion1/1
  Data Type Conversion1/1 -> Bus Creator/2  "WoWPcnt"
  Delay1/1 -> Signal Specification L/1
  Delay2/1 -> Signal Specification R/1
  Delay3/1 -> Signal Specification N/1
  Re-Encoding R/1 -> Terminator10/1  "Sim.328_MGR_DSC_Load_N"
  Re-Encoding L/1 -> Terminator9/1  "Sim.328_MGL_DSC_Load_N"
  Re-Encoding N/1 -> Terminator/1  "Sim.328_NG_DSC_Load_N"
  WOW Module/2(WOW_OUTPUT_DISABLE) -> [Sim_WOW_Output_Disable]
  Data Type Conversion2/1 -> Gain/1, Data Type Conversion/1
  Constant3/1 -> WOW Module/2(NRC_ACTIVE)
  Constant1/1 -> WOW Module/6(INITIALIZE)
  Subsystem/1(User Cmds) -> WOW Module/7(User_Cmd_In)
  WOW Module/1(Detection) -> Bus Selector/1
  WOW Module/3(NG_Out) -> Terminator1/1
  WOW Module/5(MGR_Out) -> Terminator2/1
  WOW Module/4(MGL_Out) -> Terminator3/1
  WOW Module/6(SHY_MODE) -> Terminator4/1
  WOW Module/7(User_Cmd_Out) -> Terminator5/1
  Bus Formatting NG/1(Bus Out) -> WOW Module/3(NG_In)
  Bus Formatting MGL/1(Bus Out) -> WOW Module/4(MGL_In)
  Bus Formatting MGR/1(Bus Out) -> WOW Module/5(MGR_In)
  DSC Load Conversion/1 -> Bus Formatting NG/1(WOW_N)  "Sim.NG_WOW_N"
  DSC Load Conversion/3 -> Bus Formatting MGL/1(WOW_N)  "Sim.MGL_WOW_N"
  DSC Load Conversion/5 -> Bus Formatting MGR/1(WOW_N)  "Sim.MGR_WOW_N"
  Saturation N/1 -> Re-Encoding N/1
  Saturation L/1 -> Re-Encoding L/1
  Saturation R/1 -> Re-Encoding R/1
  Bus Element In1/1 -> Load Cell and Unit Conversion/1(NG Wheel Load Lbf)
  Bus Element In4/1 -> Load Cell and Unit Conversion/2(MGL Wheel Load Lbf)
  Bus Element In5/1 -> Load Cell and Unit Conversion/3(MGR Wheel Load Lbf)
  Load Cell and Unit Conversion/1(NG Cell Load N) -> DSC Data Acquisition/1(NG Cell Load N)
  Load Cell and Unit Conversion/2(MGL Cell Load N) -> DSC Data Acquisition/2(MGL Cell Load N)
  Load Cell and Unit Conversion/3(MGR Cell Load N) -> DSC Data Acquisition/3(MGR Cell Load N)
  DSC Data Acquisition/1(NG DSC Load N) -> Delay3/1
  DSC Data Acquisition/2(MGL DSC Load N) -> Delay1/1
  DSC Data Acquisition/3(MGR DSC Load N) -> Delay2/1
  DSC Load Conversion/2 -> Terminator6/1
  DSC Load Conversion/4 -> Terminator7/1
  DSC Load Conversion/6 -> Terminator8/1

== system Lib_Piccolo/Ground Detection Systems/WoW Wrapper/Variant Subsystem/Load Cell WoW Model 23 ==
  note: Quantized DSC loads, units of N .
  note: Converted to Cell loads, units of N .
  note: Calibrated/converted Wheel loads, as used by WOW logic, units of N .
      |
      | This subsystem is auto-coded and implements signal conditioning of loads prior to use in WOW logic. Inports and Outports defined here will constitute the class interface.
  note: This subsystem is auto-coded to generate the WOW class as integrated by K2. Inports and Outports defined here will constitute the class interface.
  note: These signals are sent on the CMD and TELEM CAN Bus in the 0x3280000 ID Message
  note: Load Cell Model
  note: DSC Model
  note: K2 Data Acquisition and Processing
  note: Data Formatting for Piccolo Communications
  note: CANOpen transport delay from DSC to K2 is <1ms. Addtional delay here also accounts for worst case asynchronicity between DSC PDO and K2 sampling. Load phase delay defined in workspace.
  note: Wheel loads from FDM, units of lbf .
  note: K2 System Boundary
  Piccolo_AP_Mode : Inport
  Bus Element In5 : Inport  Port=2  PortName=WoW_Bus_In  Element=ZgrndRhLbs
  Bus Element In4 : Inport  Port=2  PortName=WoW_Bus_In  Element=ZgrndLhLbs
  Bus Element In1 : Inport  Port=2  PortName=WoW_Bus_In  Element=ZgrndNgLbs
  Bus Creator : BusCreator  Inputs=2
  Bus Selector : BusSelector  OutputSignals=CONTACT
  Bus Formatting MGL : Subsystem
  Bus Formatting MGR : Subsystem
  Bus Formatting NG : Subsystem
  Constant1 : Constant  Value=0  OutDataTypeStr=boolean
  Constant3 : Constant  Value=0  OutDataTypeStr=boolean
  DSC Data Acquisition : Subsystem
  DSC Load Conversion : $bdroot/DSC Load Conversion  SystemSampleTime=-1
  Data Type Conversion : DataTypeConversion
  Data Type Conversion1 : DataTypeConversion
  Data Type Conversion2 : DataTypeConversion  OutDataTypeStr=uint8
  Delay1 : Delay  DelayLength=SensorModel.WOW.Cell.WOWtransportDelay
  Delay2 : Delay  DelayLength=SensorModel.WOW.Cell.WOWtransportDelay
  Delay3 : Delay  DelayLength=SensorModel.WOW.Cell.WOWtransportDelay
  Gain : Gain  Gain=100
  Load Cell and Unit Conversion : Subsystem
  Re-Encoding L : Quantizer  QuantizationInterval=(SensorModel.WOW.Cell.satMaxMG-SensorModel.WOW.Cell.satMinMG)/(2^SensorModel.WOW.Cell.numBits)
  Re-Encoding N : Quantizer  QuantizationInterval=(SensorModel.WOW.Cell.satMaxNG-SensorModel.WOW.Cell.satMinNG)/(2^SensorModel.WOW.Cell.numBits)
  Re-Encoding R : Quantizer  QuantizationInterval=(SensorModel.WOW.Cell.satMaxMG-SensorModel.WOW.Cell.satMinMG)/(2^SensorModel.WOW.Cell.numBits)  LinearizeAsGain=off
  Saturation L : Saturate  UpperLimit=SensorModel.WOW.Cell.satMaxMG  LowerLimit=SensorModel.WOW.Cell.satMinMG
  Saturation N : Saturate  UpperLimit=SensorModel.WOW.Cell.satMaxNG  LowerLimit=SensorModel.WOW.Cell.satMinNG
  Saturation R : Saturate  UpperLimit=SensorModel.WOW.Cell.satMaxMG  LowerLimit=SensorModel.WOW.Cell.satMinMG
  Signal Specification L : SignalSpecification  OutDataTypeStr=single  Dimensions=[1 1]  SampleTime=dt
  Signal Specification N : SignalSpecification  OutDataTypeStr=single  Dimensions=[1 1]  SampleTime=dt
  Signal Specification R : SignalSpecification  OutDataTypeStr=single  Dimensions=[1 1]  SampleTime=dt
  Subsystem : Subsystem
  Terminator{,1..10} (11 alike) : Terminator
  WOW Module : Subsystem
  WOW_Bus_Out : Outport
  tag scope: Sim_WOW_Output_Disable=global
  wires:
  DSC Load Conversion/6 -> Terminator8/1
  DSC Load Conversion/4 -> Terminator7/1
  DSC Load Conversion/2 -> Terminator6/1
  DSC Data Acquisition/3(MGR DSC Load N) -> Delay2/1
  DSC Data Acquisition/2(MGL DSC Load N) -> Delay1/1
  DSC Data Acquisition/1(NG DSC Load N) -> Delay3/1
  Load Cell and Unit Conversion/3(MGR Cell Load N) -> DSC Data Acquisition/3(MGR Cell Load N)
  Load Cell and Unit Conversion/2(MGL Cell Load N) -> DSC Data Acquisition/2(MGL Cell Load N)
  Load Cell and Unit Conversion/1(NG Cell Load N) -> DSC Data Acquisition/1(NG Cell Load N)
  Bus Element In5/1 -> Load Cell and Unit Conversion/3(MGR Wheel Load Lbf)
  Bus Element In4/1 -> Load Cell and Unit Conversion/2(MGL Wheel Load Lbf)
  Bus Element In1/1 -> Load Cell and Unit Conversion/1(NG Wheel Load Lbf)
  Saturation R/1 -> Re-Encoding R/1
  Saturation L/1 -> Re-Encoding L/1
  Saturation N/1 -> Re-Encoding N/1
  DSC Load Conversion/5 -> Bus Formatting MGR/1(WOW_N)  "Sim.MGR_WOW_N"
  DSC Load Conversion/3 -> Bus Formatting MGL/1(WOW_N)  "Sim.MGL_WOW_N"
  DSC Load Conversion/1 -> Bus Formatting NG/1(WOW_N)  "Sim.NG_WOW_N"
  Bus Formatting MGR/1(Bus Out) -> WOW Module/5(MGR_In)
  Bus Formatting MGL/1(Bus Out) -> WOW Module/4(MGL_In)
  Bus Formatting NG/1(Bus Out) -> WOW Module/3(NG_In)
  WOW Module/7(User_Cmd_Out) -> Terminator5/1
  WOW Module/6(SHY_MODE) -> Terminator4/1
  WOW Module/4(MGL_Out) -> Terminator3/1
  WOW Module/5(MGR_Out) -> Terminator2/1
  WOW Module/3(NG_Out) -> Terminator1/1
  WOW Module/1(Detection) -> Bus Selector/1
  Subsystem/1(User Cmds) -> WOW Module/7(User_Cmd_In)
  Constant1/1 -> WOW Module/6(INITIALIZE)
  Constant3/1 -> WOW Module/2(NRC_ACTIVE)
  Data Type Conversion2/1 -> Data Type Conversion/1, Gain/1
  WOW Module/2(WOW_OUTPUT_DISABLE) -> [Sim_WOW_Output_Disable]
  Re-Encoding N/1 -> Terminator/1  "Sim.328_NG_DSC_Load_N"
  Re-Encoding L/1 -> Terminator9/1  "Sim.328_MGL_DSC_Load_N"
  Re-Encoding R/1 -> Terminator10/1  "Sim.328_MGR_DSC_Load_N"
  Delay3/1 -> Signal Specification N/1
  Delay2/1 -> Signal Specification R/1
  Delay1/1 -> Signal Specification L/1
  Data Type Conversion1/1 -> Bus Creator/2  "WoWPcnt"
  Gain/1 -> Data Type Conversion1/1
  Data Type Conversion/1 -> Bus Creator/1  "ContactBool"
  Bus Creator/1 -> WOW_Bus_Out/1
  Bus Selector/1 -> Data Type Conversion2/1  "<CONTACT>"
  Signal Specification N/1 -> Saturation N/1, DSC Load Conversion/1  "Sim.NG_DSC_Load_N"
  Signal Specification L/1 -> DSC Load Conversion/2, Saturation L/1  "Sim.MGL_DSC_Load_N"
  Signal Specification R/1 -> DSC Load Conversion/3, Saturation R/1  "Sim.MGR_DSC_Load_N"
  Piccolo_AP_Mode/1 -> WOW Module/1(PICCOLO_AP_MODE)

== system Lib_Piccolo/Ground Detection Systems/WoW Wrapper/Variant Subsystem/Load Cell WoW Model 24 ==
  note: K2 System Boundary
  note: Wheel loads from FDM, units of lbf .
  note: CANOpen transport delay from DSC to K2 is <1ms. Addtional delay here also accounts for worst case asynchronicity between DSC PDO and K2 sampling. Load phase delay defined in workspace.
  note: Data Formatting for Piccolo Communications
  note: K2 Data Acquisition and Processing
  note: DSC Model
  note: Load Cell Model
  note: These signals are sent on the CMD and TELEM CAN Bus in the 0x3280000 ID Message
  note: This subsystem is auto-coded to generate the WOW class as integrated by K2. Inports and Outports defined here will constitute the class interface.
  note: Calibrated/converted Wheel loads, as used by WOW logic, units of N .
      |
      | This subsystem is auto-coded and implements signal conditioning of loads prior to use in WOW logic. Inports and Outports defined here will constitute the class interface.
  note: Converted to Cell loads, units of N .
  note: Quantized DSC loads, units of N .
  Piccolo_AP_Mode : Inport
  Bus Element In5 : Inport  Port=2  PortName=WoW_Bus_In  Element=ZgrndRhLbs
  Bus Element In4 : Inport  Port=2  PortName=WoW_Bus_In  Element=ZgrndLhLbs
  Bus Element In1 : Inport  Port=2  PortName=WoW_Bus_In  Element=ZgrndNgLbs
  Bus Creator : BusCreator  Inputs=2
  Bus Selector : BusSelector  OutputSignals=CONTACT
  Bus Formatting MGL : Subsystem
  Bus Formatting MGR : Subsystem
  Bus Formatting NG : Subsystem
  Constant1 : Constant  Value=0  OutDataTypeStr=boolean
  Constant3 : Constant  Value=0  OutDataTypeStr=boolean
  DSC Data Acquisition : Subsystem
  DSC Load Conversion : $bdroot/DSC Load Conversion  SystemSampleTime=-1
  Data Type Conversion : DataTypeConversion
  Data Type Conversion1 : DataTypeConversion
  Data Type Conversion2 : DataTypeConversion  OutDataTypeStr=uint8
  Delay1 : Delay  DelayLength=SensorModel.WOW.Cell.WOWtransportDelay
  Delay2 : Delay  DelayLength=SensorModel.WOW.Cell.WOWtransportDelay
  Delay3 : Delay  DelayLength=SensorModel.WOW.Cell.WOWtransportDelay
  Gain : Gain  Gain=100
  Load Cell and Unit Conversion : Subsystem
  Re-Encoding L : Quantizer  QuantizationInterval=(SensorModel.WOW.Cell.satMaxMG-SensorModel.WOW.Cell.satMinMG)/(2^SensorModel.WOW.Cell.numBits)
  Re-Encoding N : Quantizer  QuantizationInterval=(SensorModel.WOW.Cell.satMaxNG-SensorModel.WOW.Cell.satMinNG)/(2^SensorModel.WOW.Cell.numBits)
  Re-Encoding R : Quantizer  QuantizationInterval=(SensorModel.WOW.Cell.satMaxMG-SensorModel.WOW.Cell.satMinMG)/(2^SensorModel.WOW.Cell.numBits)  LinearizeAsGain=off
  Saturation L : Saturate  UpperLimit=SensorModel.WOW.Cell.satMaxMG  LowerLimit=SensorModel.WOW.Cell.satMinMG
  Saturation N : Saturate  UpperLimit=SensorModel.WOW.Cell.satMaxNG  LowerLimit=SensorModel.WOW.Cell.satMinNG
  Saturation R : Saturate  UpperLimit=SensorModel.WOW.Cell.satMaxMG  LowerLimit=SensorModel.WOW.Cell.satMinMG
  Signal Specification L : SignalSpecification  OutDataTypeStr=single  Dimensions=[1 1]  SampleTime=dt
  Signal Specification N : SignalSpecification  OutDataTypeStr=single  Dimensions=[1 1]  SampleTime=dt
  Signal Specification R : SignalSpecification  OutDataTypeStr=single  Dimensions=[1 1]  SampleTime=dt
  Subsystem : Subsystem
  Terminator{,1..10} (11 alike) : Terminator
  WOW Module : Subsystem
  WOW_Bus_Out : Outport
  tag scope: Sim_WOW_Output_Disable=global
  wires:
  Piccolo_AP_Mode/1 -> WOW Module/1(PICCOLO_AP_MODE)
  Signal Specification R/1 -> Saturation R/1, DSC Load Conversion/3  "Sim.MGR_DSC_Load_N"
  Signal Specification L/1 -> Saturation L/1, DSC Load Conversion/2  "Sim.MGL_DSC_Load_N"
  Signal Specification N/1 -> DSC Load Conversion/1, Saturation N/1  "Sim.NG_DSC_Load_N"
  Bus Selector/1 -> Data Type Conversion2/1  "<CONTACT>"
  Bus Creator/1 -> WOW_Bus_Out/1
  Data Type Conversion/1 -> Bus Creator/1  "ContactBool"
  Gain/1 -> Data Type Conversion1/1
  Data Type Conversion1/1 -> Bus Creator/2  "WoWPcnt"
  Delay1/1 -> Signal Specification L/1
  Delay2/1 -> Signal Specification R/1
  Delay3/1 -> Signal Specification N/1
  Re-Encoding R/1 -> Terminator10/1  "Sim.328_MGR_DSC_Load_N"
  Re-Encoding L/1 -> Terminator9/1  "Sim.328_MGL_DSC_Load_N"
  Re-Encoding N/1 -> Terminator/1  "Sim.328_NG_DSC_Load_N"
  WOW Module/2(WOW_OUTPUT_DISABLE) -> [Sim_WOW_Output_Disable]
  Data Type Conversion2/1 -> Gain/1, Data Type Conversion/1
  Constant3/1 -> WOW Module/2(NRC_ACTIVE)
  Constant1/1 -> WOW Module/6(INITIALIZE)
  Subsystem/1(User Cmds) -> WOW Module/7(User_Cmd_In)
  WOW Module/1(Detection) -> Bus Selector/1
  WOW Module/3(NG_Out) -> Terminator1/1
  WOW Module/5(MGR_Out) -> Terminator2/1
  WOW Module/4(MGL_Out) -> Terminator3/1
  WOW Module/6(SHY_MODE) -> Terminator4/1
  WOW Module/7(User_Cmd_Out) -> Terminator5/1
  Bus Formatting NG/1(Bus Out) -> WOW Module/3(NG_In)
  Bus Formatting MGL/1(Bus Out) -> WOW Module/4(MGL_In)
  Bus Formatting MGR/1(Bus Out) -> WOW Module/5(MGR_In)
  DSC Load Conversion/1 -> Bus Formatting NG/1(WOW_N)  "Sim.NG_WOW_N"
  DSC Load Conversion/3 -> Bus Formatting MGL/1(WOW_N)  "Sim.MGL_WOW_N"
  DSC Load Conversion/5 -> Bus Formatting MGR/1(WOW_N)  "Sim.MGR_WOW_N"
  Saturation N/1 -> Re-Encoding N/1
  Saturation L/1 -> Re-Encoding L/1
  Saturation R/1 -> Re-Encoding R/1
  Bus Element In1/1 -> Load Cell and Unit Conversion/1(NG Wheel Load Lbf)
  Bus Element In4/1 -> Load Cell and Unit Conversion/2(MGL Wheel Load Lbf)
  Bus Element In5/1 -> Load Cell and Unit Conversion/3(MGR Wheel Load Lbf)
  Load Cell and Unit Conversion/1(NG Cell Load N) -> DSC Data Acquisition/1(NG Cell Load N)
  Load Cell and Unit Conversion/2(MGL Cell Load N) -> DSC Data Acquisition/2(MGL Cell Load N)
  Load Cell and Unit Conversion/3(MGR Cell Load N) -> DSC Data Acquisition/3(MGR Cell Load N)
  DSC Data Acquisition/1(NG DSC Load N) -> Delay3/1
  DSC Data Acquisition/2(MGL DSC Load N) -> Delay1/1
  DSC Data Acquisition/3(MGR DSC Load N) -> Delay2/1
  DSC Load Conversion/2 -> Terminator6/1
  DSC Load Conversion/4 -> Terminator7/1
  DSC Load Conversion/6 -> Terminator8/1

== system Lib_Piccolo/Piccolo State Machine/Landing State Machine/FlareLatch/Latch ==
  D : Inport
  Enable/!Rst : Inport  Port=2
  AND : Logic  IconShape=distinctive  AllPortsSameDT=off  OutDataTypeStr=boolean
  Constant : Constant
  OR : Logic  Operator=OR  IconShape=distinctive  AllPortsSameDT=off  OutDataTypeStr=boolean
  Switch : Switch  Criteria=u2 > Threshold  Threshold=0.5
  Unit Delay : UnitDelay  SampleTime=-1
  Q_Latched : Outport
  wires:
  Unit Delay/1 -> OR/2
  Switch/1 -> Q_Latched/1, Unit Delay/1
  D/1 -> Switch/3, OR/1
  OR/1 -> AND/1
  AND/1 -> Switch/2
  Enable/!Rst/1 -> AND/2
  Constant/1 -> Switch/1

== system Lib_Piccolo/Pitch to Elevator/Reference Frame Conversion and Pitch Rate Limit Determination/AeroVsStruct_Limit/Flap Compensation ==
  CL_Limit_in : Inport
  Gain : Gain  Gain=dCl_per_dFlap
  Sum : Sum  Inputs=|++
  CL_Limit_adjusted : Outport
  wires:
  [flapCmd] -> Gain/1
  Gain/1 -> Sum/2
  Sum/1 -> CL_Limit_adjusted/1
  CL_Limit_in/1 -> Sum/1
